simulink model "SimulinkObserver"  (R2016b)
settings: Solver=VariableStepAuto  StartTime=0.0  StopTime=5  RelTol=1e-3
undefined symbols (not defined in the file): A, B, C, K, Kf
settings Model: Creator=kwstas  LastModifiedBy=kwstas
settings SolverCC: MaxConsecutiveZCs=10000

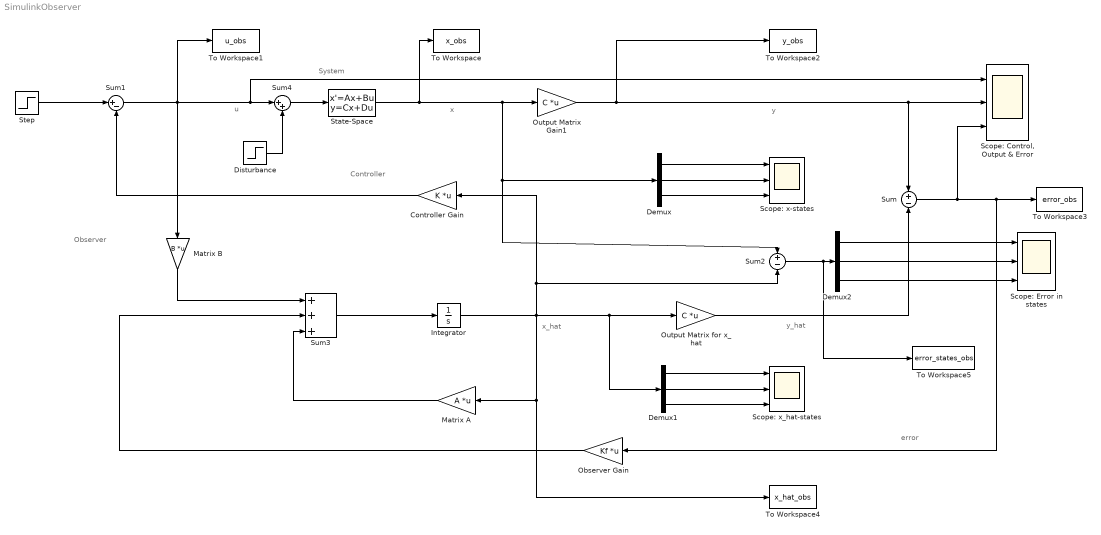
== system SimulinkObserver ==
  note: Observer
  note: Controller
  note: System
  note: y_hat
  note: error
  note: y
  note: u
  note: x_hat
  note: x
  Controller Gain : Gain  Gain=K  Multiplication=Matrix(K*u) (u vector)
  Demux : Demux  Outputs=3
  Demux1 : Demux  Outputs=3
  Demux2 : Demux  Outputs=3
  Disturbance : Step  After=3  SampleTime=0
  Integrator : Integrator
  Matrix A : Gain  Gain=A  Multiplication=Matrix(K*u) (u vector)
  Matrix B : Gain  Gain=B  Multiplication=Matrix(K*u) (u vector)
  Observer Gain : Gain  Gain=Kf  Multiplication=Matrix(K*u) (u vector)
  Output Matrix Gain1 : Gain  Gain=C  Multiplication=Matrix(K*u) (u vector)
  Output Matrix for x_hat : Gain  Gain=C  Multiplication=Matrix(K*u) (u vector)
  "Scope: Control, Output & Error" : Scope  NumInputPorts=3
  Scope: Error in states : Scope  NumInputPorts=3
  Scope: x-states : Scope  NumInputPorts=3
  Scope: x_hat-states : Scope  NumInputPorts=3
  State-Space : StateSpace  A=A  B=B  C=eye(length(A))  D=[0;0;0]  X0=[0;0;0]
  Step : Step  Time=0  After=0  SampleTime=0
  Sum : Sum  Inputs=+-
  Sum1 : Sum  Inputs=|+-
  Sum2 : Sum  Inputs=+-
  Sum3 : Sum  Inputs=3
  Sum4 : Sum  Inputs=|++
  To Workspace : ToWorkspace  VariableName=x_obs  SaveFormat=Timeseries  SampleTime=-1
  To Workspace1 : ToWorkspace  VariableName=u_obs  SaveFormat=Timeseries  SampleTime=-1
  To Workspace2 : ToWorkspace  VariableName=y_obs  SaveFormat=Timeseries  SampleTime=-1
  To Workspace3 : ToWorkspace  VariableName=error_obs  SaveFormat=Timeseries  SampleTime=-1
  To Workspace4 : ToWorkspace  VariableName=x_hat_obs  SaveFormat=Timeseries  SampleTime=-1
  To Workspace5 : ToWorkspace  VariableName=error_states_obs  SaveFormat=Timeseries  SampleTime=-1
  wires:
  Step/1 -> Sum1/1
  State-Space/1 -> To Workspace/1, Sum2/1, Demux/1, Output Matrix Gain1/1
  Sum3/1 -> Integrator/1
  Integrator/1 -> Demux1/1, Output Matrix for x_hat/1, To Workspace4/1, Matrix A/1, Sum2/2, Controller Gain/1
  Controller Gain/1 -> Sum1/2
  Matrix B/1 -> Sum3/1
  Matrix A/1 -> Sum3/3
  Sum/1 -> "Scope: Control, Output & Error"/3, To Workspace3/1, Observer Gain/1
  Observer Gain/1 -> Sum3/2
  Demux/2 -> Scope: x-states/2
  Demux/3 -> Scope: x-states/3
  Demux/1 -> Scope: x-states/1
  Sum1/1 -> Sum4/1, "Scope: Control, Output & Error"/1, Matrix B/1, To Workspace1/1
  Demux1/1 -> Scope: x_hat-states/1
  Demux1/2 -> Scope: x_hat-states/2
  Demux1/3 -> Scope: x_hat-states/3
  Sum2/1 -> To Workspace5/1, Demux2/1
  Demux2/2 -> Scope: Error in states/2
  Demux2/3 -> Scope: Error in states/3
  Demux2/1 -> Scope: Error in states/1
  Output Matrix for x_hat/1 -> Sum/2
  Sum4/1 -> State-Space/1
  Disturbance/1 -> Sum4/2
  Output Matrix Gain1/1 -> Sum/1, "Scope: Control, Output & Error"/2, To Workspace2/1
